simulink model "TrajectoryGenerator2DOF_freq"  (R2023b)
settings: Solver=FixedStepDiscrete  StartTime=0.0  StopTime=1.2*1.4  FixedStep=0.002  RelTol=1e-3
undefined symbols (not defined in the file or in its folder): M_z, Smoothers, Ts
(part 2 of 2)

== system TrajectoryGenerator2DOF_freq/Trajectory Generator4/M12 ==
  x : Inport
  Discrete FIR Filter1 : DiscreteFir  Coefficients=1/N/Ts*[1 zeros(1,N-1) -1]  InitialStates=Q0  SampleTime=Ts
  Discrete Filter : DiscreteFilter  Numerator=[0 Ts]  Denominator=[1 -1]  InitialStates=Q0  SampleTime=Ts
  y : Outport
  dy : Outport  Port=2
  wires:
  Discrete FIR Filter1/1 -> Discrete Filter/1, dy/1
  x/1 -> Discrete FIR Filter1/1
  Discrete Filter/1 -> y/1

== system TrajectoryGenerator2DOF_freq/Trajectory Generator4/M13 ==
  x : Inport
  Discrete FIR Filter1 : DiscreteFir  Coefficients=1/N/Ts*[1 zeros(1,N-1) -1]  InitialStates=Q0  SampleTime=Ts
  Discrete Filter : DiscreteFilter  Numerator=[0 Ts]  Denominator=[1 -1]  InitialStates=Q0  SampleTime=Ts
  y : Outport
  dy : Outport  Port=2
  wires:
  Discrete FIR Filter1/1 -> Discrete Filter/1, dy/1
  x/1 -> Discrete FIR Filter1/1
  Discrete Filter/1 -> y/1

== system TrajectoryGenerator2DOF_freq/Trajectory Generator4/M14 ==
  x : Inport
  Discrete FIR Filter1 : DiscreteFir  Coefficients=1/N/Ts*[1 zeros(1,N-1) -1]  InitialStates=Q0  SampleTime=Ts
  Discrete Filter : DiscreteFilter  Numerator=[0 Ts]  Denominator=[1 -1]  InitialStates=Q0  SampleTime=Ts
  y : Outport
  dy : Outport  Port=2
  wires:
  Discrete FIR Filter1/1 -> Discrete Filter/1, dy/1
  x/1 -> Discrete FIR Filter1/1
  Discrete Filter/1 -> y/1

== system TrajectoryGenerator2DOF_freq/Trajectory Generator4/M22 ==
  x : Inport
  Discrete FIR Filter1 : DiscreteFir  Coefficients=1/N/Ts*[1 zeros(1,N-1) -1]  InitialStates=Q0  SampleTime=Ts
  Discrete Filter : DiscreteFilter  Numerator=[0 Ts]  Denominator=[1 -1]  InitialStates=Q0  SampleTime=Ts
  y : Outport
  dy : Outport  Port=2
  wires:
  Discrete FIR Filter1/1 -> Discrete Filter/1, dy/1
  x/1 -> Discrete FIR Filter1/1
  Discrete Filter/1 -> y/1

== system TrajectoryGenerator2DOF_freq/Trajectory Generator4/M23 ==
  x : Inport
  Discrete FIR Filter1 : DiscreteFir  Coefficients=1/N/Ts*[1 zeros(1,N-1) -1]  InitialStates=Q0  SampleTime=Ts
  Discrete Filter : DiscreteFilter  Numerator=[0 Ts]  Denominator=[1 -1]  InitialStates=Q0  SampleTime=Ts
  y : Outport
  dy : Outport  Port=2
  wires:
  Discrete FIR Filter1/1 -> Discrete Filter/1, dy/1
  x/1 -> Discrete FIR Filter1/1
  Discrete Filter/1 -> y/1

== system TrajectoryGenerator2DOF_freq/Trajectory Generator4/M24 ==
  x : Inport
  Discrete FIR Filter1 : DiscreteFir  Coefficients=1/N/Ts*[1 zeros(1,N-1) -1]  InitialStates=Q0  SampleTime=Ts
  Discrete Filter : DiscreteFilter  Numerator=[0 Ts]  Denominator=[1 -1]  InitialStates=Q0  SampleTime=Ts
  y : Outport
  dy : Outport  Port=2
  wires:
  Discrete FIR Filter1/1 -> Discrete Filter/1, dy/1
  x/1 -> Discrete FIR Filter1/1
  Discrete Filter/1 -> y/1

== system TrajectoryGenerator2DOF_freq/Trajectory Generator4/M33 ==
  x : Inport
  Discrete FIR Filter1 : DiscreteFir  Coefficients=1/N/Ts*[1 zeros(1,N-1) -1]  InitialStates=Q0  SampleTime=Ts
  Discrete Filter : DiscreteFilter  Numerator=[0 Ts]  Denominator=[1 -1]  InitialStates=Q0  SampleTime=Ts
  y : Outport
  dy : Outport  Port=2
  wires:
  Discrete FIR Filter1/1 -> Discrete Filter/1, dy/1
  x/1 -> Discrete FIR Filter1/1
  Discrete Filter/1 -> y/1

== system TrajectoryGenerator2DOF_freq/Trajectory Generator4/M34 ==
  x : Inport
  Discrete FIR Filter1 : DiscreteFir  Coefficients=1/N/Ts*[1 zeros(1,N-1) -1]  InitialStates=Q0  SampleTime=Ts
  Discrete Filter : DiscreteFilter  Numerator=[0 Ts]  Denominator=[1 -1]  InitialStates=Q0  SampleTime=Ts
  y : Outport
  dy : Outport  Port=2
  wires:
  Discrete FIR Filter1/1 -> Discrete Filter/1, dy/1
  x/1 -> Discrete FIR Filter1/1
  Discrete Filter/1 -> y/1

== system TrajectoryGenerator2DOF_freq/Trajectory Generator4/M44 ==
  x : Inport
  Discrete FIR Filter1 : DiscreteFir  Coefficients=1/N/Ts*[1 zeros(1,N-1) -1]  InitialStates=Q0  SampleTime=Ts
  Discrete Filter : DiscreteFilter  Numerator=[0 Ts]  Denominator=[1 -1]  InitialStates=Q0  SampleTime=Ts
  y : Outport
  dy : Outport  Port=2
  wires:
  Discrete FIR Filter1/1 -> Discrete Filter/1, dy/1
  x/1 -> Discrete FIR Filter1/1
  Discrete Filter/1 -> y/1

== system TrajectoryGenerator2DOF_freq/Trajectory Generator5/M11 ==
  x : Inport
  Discrete FIR Filter1 : DiscreteFir  Coefficients=1/N/Ts*[1 zeros(1,N-1) -1]  InitialStates=Q0  SampleTime=Ts
  Discrete Filter : DiscreteFilter  Numerator=[0 Ts]  Denominator=[1 -1]  InitialStates=Q0  SampleTime=Ts
  y : Outport
  dy : Outport  Port=2
  wires:
  Discrete FIR Filter1/1 -> Discrete Filter/1, dy/1
  x/1 -> Discrete FIR Filter1/1
  Discrete Filter/1 -> y/1

== system TrajectoryGenerator2DOF_freq/Trajectory Generator5/M12 ==
  x : Inport
  Discrete FIR Filter1 : DiscreteFir  Coefficients=1/N/Ts*[1 zeros(1,N-1) -1]  InitialStates=Q0  SampleTime=Ts
  Discrete Filter : DiscreteFilter  Numerator=[0 Ts]  Denominator=[1 -1]  InitialStates=Q0  SampleTime=Ts
  y : Outport
  dy : Outport  Port=2
  wires:
  Discrete FIR Filter1/1 -> Discrete Filter/1, dy/1
  x/1 -> Discrete FIR Filter1/1
  Discrete Filter/1 -> y/1

== system TrajectoryGenerator2DOF_freq/Trajectory Generator5/M13 ==
  x : Inport
  Discrete FIR Filter1 : DiscreteFir  Coefficients=1/N/Ts*[1 zeros(1,N-1) -1]  InitialStates=Q0  SampleTime=Ts
  Discrete Filter : DiscreteFilter  Numerator=[0 Ts]  Denominator=[1 -1]  InitialStates=Q0  SampleTime=Ts
  y : Outport
  dy : Outport  Port=2
  wires:
  Discrete FIR Filter1/1 -> Discrete Filter/1, dy/1
  x/1 -> Discrete FIR Filter1/1
  Discrete Filter/1 -> y/1

== system TrajectoryGenerator2DOF_freq/Trajectory Generator5/M14 ==
  x : Inport
  Discrete FIR Filter1 : DiscreteFir  Coefficients=1/N/Ts*[1 zeros(1,N-1) -1]  InitialStates=Q0  SampleTime=Ts
  Discrete Filter : DiscreteFilter  Numerator=[0 Ts]  Denominator=[1 -1]  InitialStates=Q0  SampleTime=Ts
  y : Outport
  dy : Outport  Port=2
  wires:
  Discrete FIR Filter1/1 -> Discrete Filter/1, dy/1
  x/1 -> Discrete FIR Filter1/1
  Discrete Filter/1 -> y/1

== system TrajectoryGenerator2DOF_freq/Trajectory Generator5/M22 ==
  x : Inport
  Discrete FIR Filter1 : DiscreteFir  Coefficients=1/N/Ts*[1 zeros(1,N-1) -1]  InitialStates=Q0  SampleTime=Ts
  Discrete Filter : DiscreteFilter  Numerator=[0 Ts]  Denominator=[1 -1]  InitialStates=Q0  SampleTime=Ts
  y : Outport
  dy : Outport  Port=2
  wires:
  Discrete FIR Filter1/1 -> Discrete Filter/1, dy/1
  x/1 -> Discrete FIR Filter1/1
  Discrete Filter/1 -> y/1

== system TrajectoryGenerator2DOF_freq/Trajectory Generator5/M23 ==
  x : Inport
  Discrete FIR Filter1 : DiscreteFir  Coefficients=1/N/Ts*[1 zeros(1,N-1) -1]  InitialStates=Q0  SampleTime=Ts
  Discrete Filter : DiscreteFilter  Numerator=[0 Ts]  Denominator=[1 -1]  InitialStates=Q0  SampleTime=Ts
  y : Outport
  dy : Outport  Port=2
  wires:
  Discrete FIR Filter1/1 -> Discrete Filter/1, dy/1
  x/1 -> Discrete FIR Filter1/1
  Discrete Filter/1 -> y/1

== system TrajectoryGenerator2DOF_freq/Trajectory Generator5/M24 ==
  x : Inport
  Discrete FIR Filter1 : DiscreteFir  Coefficients=1/N/Ts*[1 zeros(1,N-1) -1]  InitialStates=Q0  SampleTime=Ts
  Discrete Filter : DiscreteFilter  Numerator=[0 Ts]  Denominator=[1 -1]  InitialStates=Q0  SampleTime=Ts
  y : Outport
  dy : Outport  Port=2
  wires:
  Discrete FIR Filter1/1 -> Discrete Filter/1, dy/1
  x/1 -> Discrete FIR Filter1/1
  Discrete Filter/1 -> y/1

== system TrajectoryGenerator2DOF_freq/Trajectory Generator5/M33 ==
  x : Inport
  Discrete FIR Filter1 : DiscreteFir  Coefficients=1/N/Ts*[1 zeros(1,N-1) -1]  InitialStates=Q0  SampleTime=Ts
  Discrete Filter : DiscreteFilter  Numerator=[0 Ts]  Denominator=[1 -1]  InitialStates=Q0  SampleTime=Ts
  y : Outport
  dy : Outport  Port=2
  wires:
  Discrete FIR Filter1/1 -> Discrete Filter/1, dy/1
  x/1 -> Discrete FIR Filter1/1
  Discrete Filter/1 -> y/1

== system TrajectoryGenerator2DOF_freq/Trajectory Generator5/M34 ==
  x : Inport
  Discrete FIR Filter1 : DiscreteFir  Coefficients=1/N/Ts*[1 zeros(1,N-1) -1]  InitialStates=Q0  SampleTime=Ts
  Discrete Filter : DiscreteFilter  Numerator=[0 Ts]  Denominator=[1 -1]  InitialStates=Q0  SampleTime=Ts
  y : Outport
  dy : Outport  Port=2
  wires:
  Discrete FIR Filter1/1 -> Discrete Filter/1, dy/1
  x/1 -> Discrete FIR Filter1/1
  Discrete Filter/1 -> y/1

== system TrajectoryGenerator2DOF_freq/Trajectory Generator5/M44 ==
  x : Inport
  Discrete FIR Filter1 : DiscreteFir  Coefficients=1/N/Ts*[1 zeros(1,N-1) -1]  InitialStates=Q0  SampleTime=Ts
  Discrete Filter : DiscreteFilter  Numerator=[0 Ts]  Denominator=[1 -1]  InitialStates=Q0  SampleTime=Ts
  y : Outport
  dy : Outport  Port=2
  wires:
  Discrete FIR Filter1/1 -> Discrete Filter/1, dy/1
  x/1 -> Discrete FIR Filter1/1
  Discrete Filter/1 -> y/1

== system TrajectoryGenerator2DOF_freq/Trajectory Generator6/M11 ==
  x : Inport
  Discrete FIR Filter1 : DiscreteFir  Coefficients=1/N/Ts*[1 zeros(1,N-1) -1]  InitialStates=Q0  SampleTime=Ts
  Discrete Filter : DiscreteFilter  Numerator=[0 Ts]  Denominator=[1 -1]  InitialStates=Q0  SampleTime=Ts
  y : Outport
  dy : Outport  Port=2
  wires:
  Discrete FIR Filter1/1 -> Discrete Filter/1, dy/1
  x/1 -> Discrete FIR Filter1/1
  Discrete Filter/1 -> y/1

== system TrajectoryGenerator2DOF_freq/Trajectory Generator6/M12 ==
  x : Inport
  Discrete FIR Filter1 : DiscreteFir  Coefficients=1/N/Ts*[1 zeros(1,N-1) -1]  InitialStates=Q0  SampleTime=Ts
  Discrete Filter : DiscreteFilter  Numerator=[0 Ts]  Denominator=[1 -1]  InitialStates=Q0  SampleTime=Ts
  y : Outport
  dy : Outport  Port=2
  wires:
  Discrete FIR Filter1/1 -> Discrete Filter/1, dy/1
  x/1 -> Discrete FIR Filter1/1
  Discrete Filter/1 -> y/1

== system TrajectoryGenerator2DOF_freq/Trajectory Generator6/M13 ==
  x : Inport
  Discrete FIR Filter1 : DiscreteFir  Coefficients=1/N/Ts*[1 zeros(1,N-1) -1]  InitialStates=Q0  SampleTime=Ts
  Discrete Filter : DiscreteFilter  Numerator=[0 Ts]  Denominator=[1 -1]  InitialStates=Q0  SampleTime=Ts
  y : Outport
  dy : Outport  Port=2
  wires:
  Discrete FIR Filter1/1 -> Discrete Filter/1, dy/1
  x/1 -> Discrete FIR Filter1/1
  Discrete Filter/1 -> y/1

== system TrajectoryGenerator2DOF_freq/Trajectory Generator6/M14 ==
  x : Inport
  Discrete FIR Filter1 : DiscreteFir  Coefficients=1/N/Ts*[1 zeros(1,N-1) -1]  InitialStates=Q0  SampleTime=Ts
  Discrete Filter : DiscreteFilter  Numerator=[0 Ts]  Denominator=[1 -1]  InitialStates=Q0  SampleTime=Ts
  y : Outport
  dy : Outport  Port=2
  wires:
  Discrete FIR Filter1/1 -> Discrete Filter/1, dy/1
  x/1 -> Discrete FIR Filter1/1
  Discrete Filter/1 -> y/1

== system TrajectoryGenerator2DOF_freq/Trajectory Generator6/M22 ==
  x : Inport
  Discrete FIR Filter1 : DiscreteFir  Coefficients=1/N/Ts*[1 zeros(1,N-1) -1]  InitialStates=Q0  SampleTime=Ts
  Discrete Filter : DiscreteFilter  Numerator=[0 Ts]  Denominator=[1 -1]  InitialStates=Q0  SampleTime=Ts
  y : Outport
  dy : Outport  Port=2
  wires:
  Discrete FIR Filter1/1 -> Discrete Filter/1, dy/1
  x/1 -> Discrete FIR Filter1/1
  Discrete Filter/1 -> y/1

== system TrajectoryGenerator2DOF_freq/Trajectory Generator6/M23 ==
  x : Inport
  Discrete FIR Filter1 : DiscreteFir  Coefficients=1/N/Ts*[1 zeros(1,N-1) -1]  InitialStates=Q0  SampleTime=Ts
  Discrete Filter : DiscreteFilter  Numerator=[0 Ts]  Denominator=[1 -1]  InitialStates=Q0  SampleTime=Ts
  y : Outport
  dy : Outport  Port=2
  wires:
  Discrete FIR Filter1/1 -> Discrete Filter/1, dy/1
  x/1 -> Discrete FIR Filter1/1
  Discrete Filter/1 -> y/1

== system TrajectoryGenerator2DOF_freq/Trajectory Generator6/M24 ==
  x : Inport
  Discrete FIR Filter1 : DiscreteFir  Coefficients=1/N/Ts*[1 zeros(1,N-1) -1]  InitialStates=Q0  SampleTime=Ts
  Discrete Filter : DiscreteFilter  Numerator=[0 Ts]  Denominator=[1 -1]  InitialStates=Q0  SampleTime=Ts
  y : Outport
  dy : Outport  Port=2
  wires:
  Discrete FIR Filter1/1 -> Discrete Filter/1, dy/1
  x/1 -> Discrete FIR Filter1/1
  Discrete Filter/1 -> y/1

== system TrajectoryGenerator2DOF_freq/Trajectory Generator6/M33 ==
  x : Inport
  Discrete FIR Filter1 : DiscreteFir  Coefficients=1/N/Ts*[1 zeros(1,N-1) -1]  InitialStates=Q0  SampleTime=Ts
  Discrete Filter : DiscreteFilter  Numerator=[0 Ts]  Denominator=[1 -1]  InitialStates=Q0  SampleTime=Ts
  y : Outport
  dy : Outport  Port=2
  wires:
  Discrete FIR Filter1/1 -> Discrete Filter/1, dy/1
  x/1 -> Discrete FIR Filter1/1
  Discrete Filter/1 -> y/1

== system TrajectoryGenerator2DOF_freq/Trajectory Generator6/M34 ==
  x : Inport
  Discrete FIR Filter1 : DiscreteFir  Coefficients=1/N/Ts*[1 zeros(1,N-1) -1]  InitialStates=Q0  SampleTime=Ts
  Discrete Filter : DiscreteFilter  Numerator=[0 Ts]  Denominator=[1 -1]  InitialStates=Q0  SampleTime=Ts
  y : Outport
  dy : Outport  Port=2
  wires:
  Discrete FIR Filter1/1 -> Discrete Filter/1, dy/1
  x/1 -> Discrete FIR Filter1/1
  Discrete Filter/1 -> y/1

== system TrajectoryGenerator2DOF_freq/Trajectory Generator6/M44 ==
  x : Inport
  Discrete FIR Filter1 : DiscreteFir  Coefficients=1/N/Ts*[1 zeros(1,N-1) -1]  InitialStates=Q0  SampleTime=Ts
  Discrete Filter : DiscreteFilter  Numerator=[0 Ts]  Denominator=[1 -1]  InitialStates=Q0  SampleTime=Ts
  y : Outport
  dy : Outport  Port=2
  wires:
  Discrete FIR Filter1/1 -> Discrete Filter/1, dy/1
  x/1 -> Discrete FIR Filter1/1
  Discrete Filter/1 -> y/1

== system TrajectoryGenerator2DOF_freq/Trajectory Generator7/M11 ==
  x : Inport
  Discrete FIR Filter1 : DiscreteFir  Coefficients=1/N/Ts*[1 zeros(1,N-1) -1]  InitialStates=Q0  SampleTime=Ts
  Discrete Filter : DiscreteFilter  Numerator=[0 Ts]  Denominator=[1 -1]  InitialStates=Q0  SampleTime=Ts
  y : Outport
  dy : Outport  Port=2
  wires:
  Discrete FIR Filter1/1 -> Discrete Filter/1, dy/1
  x/1 -> Discrete FIR Filter1/1
  Discrete Filter/1 -> y/1

== system TrajectoryGenerator2DOF_freq/Trajectory Generator7/M12 ==
  x : Inport
  Discrete FIR Filter1 : DiscreteFir  Coefficients=1/N/Ts*[1 zeros(1,N-1) -1]  InitialStates=Q0  SampleTime=Ts
  Discrete Filter : DiscreteFilter  Numerator=[0 Ts]  Denominator=[1 -1]  InitialStates=Q0  SampleTime=Ts
  y : Outport
  dy : Outport  Port=2
  wires:
  Discrete FIR Filter1/1 -> Discrete Filter/1, dy/1
  x/1 -> Discrete FIR Filter1/1
  Discrete Filter/1 -> y/1

== system TrajectoryGenerator2DOF_freq/Trajectory Generator7/M13 ==
  x : Inport
  Discrete FIR Filter1 : DiscreteFir  Coefficients=1/N/Ts*[1 zeros(1,N-1) -1]  InitialStates=Q0  SampleTime=Ts
  Discrete Filter : DiscreteFilter  Numerator=[0 Ts]  Denominator=[1 -1]  InitialStates=Q0  SampleTime=Ts
  y : Outport
  dy : Outport  Port=2
  wires:
  Discrete FIR Filter1/1 -> Discrete Filter/1, dy/1
  x/1 -> Discrete FIR Filter1/1
  Discrete Filter/1 -> y/1

== system TrajectoryGenerator2DOF_freq/Trajectory Generator7/M14 ==
  x : Inport
  Discrete FIR Filter1 : DiscreteFir  Coefficients=1/N/Ts*[1 zeros(1,N-1) -1]  InitialStates=Q0  SampleTime=Ts
  Discrete Filter : DiscreteFilter  Numerator=[0 Ts]  Denominator=[1 -1]  InitialStates=Q0  SampleTime=Ts
  y : Outport
  dy : Outport  Port=2
  wires:
  Discrete FIR Filter1/1 -> Discrete Filter/1, dy/1
  x/1 -> Discrete FIR Filter1/1
  Discrete Filter/1 -> y/1

== system TrajectoryGenerator2DOF_freq/Trajectory Generator7/M22 ==
  x : Inport
  Discrete FIR Filter1 : DiscreteFir  Coefficients=1/N/Ts*[1 zeros(1,N-1) -1]  InitialStates=Q0  SampleTime=Ts
  Discrete Filter : DiscreteFilter  Numerator=[0 Ts]  Denominator=[1 -1]  InitialStates=Q0  SampleTime=Ts
  y : Outport
  dy : Outport  Port=2
  wires:
  Discrete FIR Filter1/1 -> Discrete Filter/1, dy/1
  x/1 -> Discrete FIR Filter1/1
  Discrete Filter/1 -> y/1

== system TrajectoryGenerator2DOF_freq/Trajectory Generator7/M23 ==
  x : Inport
  Discrete FIR Filter1 : DiscreteFir  Coefficients=1/N/Ts*[1 zeros(1,N-1) -1]  InitialStates=Q0  SampleTime=Ts
  Discrete Filter : DiscreteFilter  Numerator=[0 Ts]  Denominator=[1 -1]  InitialStates=Q0  SampleTime=Ts
  y : Outport
  dy : Outport  Port=2
  wires:
  Discrete FIR Filter1/1 -> Discrete Filter/1, dy/1
  x/1 -> Discrete FIR Filter1/1
  Discrete Filter/1 -> y/1

== system TrajectoryGenerator2DOF_freq/Trajectory Generator7/M24 ==
  x : Inport
  Discrete FIR Filter1 : DiscreteFir  Coefficients=1/N/Ts*[1 zeros(1,N-1) -1]  InitialStates=Q0  SampleTime=Ts
  Discrete Filter : DiscreteFilter  Numerator=[0 Ts]  Denominator=[1 -1]  InitialStates=Q0  SampleTime=Ts
  y : Outport
  dy : Outport  Port=2
  wires:
  Discrete FIR Filter1/1 -> Discrete Filter/1, dy/1
  x/1 -> Discrete FIR Filter1/1
  Discrete Filter/1 -> y/1

== system TrajectoryGenerator2DOF_freq/Trajectory Generator7/M33 ==
  x : Inport
  Discrete FIR Filter1 : DiscreteFir  Coefficients=1/N/Ts*[1 zeros(1,N-1) -1]  InitialStates=Q0  SampleTime=Ts
  Discrete Filter : DiscreteFilter  Numerator=[0 Ts]  Denominator=[1 -1]  InitialStates=Q0  SampleTime=Ts
  y : Outport
  dy : Outport  Port=2
  wires:
  Discrete FIR Filter1/1 -> Discrete Filter/1, dy/1
  x/1 -> Discrete FIR Filter1/1
  Discrete Filter/1 -> y/1

== system TrajectoryGenerator2DOF_freq/Trajectory Generator7/M34 ==
  x : Inport
  Discrete FIR Filter1 : DiscreteFir  Coefficients=1/N/Ts*[1 zeros(1,N-1) -1]  InitialStates=Q0  SampleTime=Ts
  Discrete Filter : DiscreteFilter  Numerator=[0 Ts]  Denominator=[1 -1]  InitialStates=Q0  SampleTime=Ts
  y : Outport
  dy : Outport  Port=2
  wires:
  Discrete FIR Filter1/1 -> Discrete Filter/1, dy/1
  x/1 -> Discrete FIR Filter1/1
  Discrete Filter/1 -> y/1

== system TrajectoryGenerator2DOF_freq/Trajectory Generator7/M44 ==
  x : Inport
  Discrete FIR Filter1 : DiscreteFir  Coefficients=1/N/Ts*[1 zeros(1,N-1) -1]  InitialStates=Q0  SampleTime=Ts
  Discrete Filter : DiscreteFilter  Numerator=[0 Ts]  Denominator=[1 -1]  InitialStates=Q0  SampleTime=Ts
  y : Outport
  dy : Outport  Port=2
  wires:
  Discrete FIR Filter1/1 -> Discrete Filter/1, dy/1
  x/1 -> Discrete FIR Filter1/1
  Discrete Filter/1 -> y/1

== system TrajectoryGenerator2DOF_freq/Trajectory Generator8/M11 ==
  x : Inport
  Discrete FIR Filter1 : DiscreteFir  Coefficients=1/N/Ts*[1 zeros(1,N-1) -1]  InitialStates=Q0  SampleTime=Ts
  Discrete Filter : DiscreteFilter  Numerator=[0 Ts]  Denominator=[1 -1]  InitialStates=Q0  SampleTime=Ts
  y : Outport
  dy : Outport  Port=2
  wires:
  Discrete FIR Filter1/1 -> Discrete Filter/1, dy/1
  x/1 -> Discrete FIR Filter1/1
  Discrete Filter/1 -> y/1

== system TrajectoryGenerator2DOF_freq/Trajectory Generator8/M12 ==
  x : Inport
  Discrete FIR Filter1 : DiscreteFir  Coefficients=1/N/Ts*[1 zeros(1,N-1) -1]  InitialStates=Q0  SampleTime=Ts
  Discrete Filter : DiscreteFilter  Numerator=[0 Ts]  Denominator=[1 -1]  InitialStates=Q0  SampleTime=Ts
  y : Outport
  dy : Outport  Port=2
  wires:
  Discrete FIR Filter1/1 -> Discrete Filter/1, dy/1
  x/1 -> Discrete FIR Filter1/1
  Discrete Filter/1 -> y/1

== system TrajectoryGenerator2DOF_freq/Trajectory Generator8/M13 ==
  x : Inport
  Discrete FIR Filter1 : DiscreteFir  Coefficients=1/N/Ts*[1 zeros(1,N-1) -1]  InitialStates=Q0  SampleTime=Ts
  Discrete Filter : DiscreteFilter  Numerator=[0 Ts]  Denominator=[1 -1]  InitialStates=Q0  SampleTime=Ts
  y : Outport
  dy : Outport  Port=2
  wires:
  Discrete FIR Filter1/1 -> Discrete Filter/1, dy/1
  x/1 -> Discrete FIR Filter1/1
  Discrete Filter/1 -> y/1

== system TrajectoryGenerator2DOF_freq/Trajectory Generator8/M14 ==
  x : Inport
  Discrete FIR Filter1 : DiscreteFir  Coefficients=1/N/Ts*[1 zeros(1,N-1) -1]  InitialStates=Q0  SampleTime=Ts
  Discrete Filter : DiscreteFilter  Numerator=[0 Ts]  Denominator=[1 -1]  InitialStates=Q0  SampleTime=Ts
  y : Outport
  dy : Outport  Port=2
  wires:
  Discrete FIR Filter1/1 -> Discrete Filter/1, dy/1
  x/1 -> Discrete FIR Filter1/1
  Discrete Filter/1 -> y/1

== system TrajectoryGenerator2DOF_freq/Trajectory Generator8/M15 ==
  x : Inport
  Discrete FIR Filter1 : DiscreteFir  Coefficients=1/N/Ts*[1 zeros(1,N-1) -1]  InitialStates=Q0  SampleTime=Ts
  Discrete Filter : DiscreteFilter  Numerator=[0 Ts]  Denominator=[1 -1]  InitialStates=Q0  SampleTime=Ts
  y : Outport
  dy : Outport  Port=2
  wires:
  Discrete FIR Filter1/1 -> Discrete Filter/1, dy/1
  x/1 -> Discrete FIR Filter1/1
  Discrete Filter/1 -> y/1

== system TrajectoryGenerator2DOF_freq/Trajectory Generator8/M16 ==
  x : Inport
  Discrete FIR Filter1 : DiscreteFir  Coefficients=1/N/Ts*[1 zeros(1,N-1) -1]  InitialStates=Q0  SampleTime=Ts
  Discrete Filter : DiscreteFilter  Numerator=[0 Ts]  Denominator=[1 -1]  InitialStates=Q0  SampleTime=Ts
  y : Outport
  dy : Outport  Port=2
  wires:
  Discrete FIR Filter1/1 -> Discrete Filter/1, dy/1
  x/1 -> Discrete FIR Filter1/1
  Discrete Filter/1 -> y/1

== system TrajectoryGenerator2DOF_freq/Trajectory Generator8/M22 ==
  x : Inport
  Discrete FIR Filter1 : DiscreteFir  Coefficients=1/N/Ts*[1 zeros(1,N-1) -1]  InitialStates=Q0  SampleTime=Ts
  Discrete Filter : DiscreteFilter  Numerator=[0 Ts]  Denominator=[1 -1]  InitialStates=Q0  SampleTime=Ts
  y : Outport
  dy : Outport  Port=2
  wires:
  Discrete FIR Filter1/1 -> Discrete Filter/1, dy/1
  x/1 -> Discrete FIR Filter1/1
  Discrete Filter/1 -> y/1

== system TrajectoryGenerator2DOF_freq/Trajectory Generator8/M23 ==
  x : Inport
  Discrete FIR Filter1 : DiscreteFir  Coefficients=1/N/Ts*[1 zeros(1,N-1) -1]  InitialStates=Q0  SampleTime=Ts
  Discrete Filter : DiscreteFilter  Numerator=[0 Ts]  Denominator=[1 -1]  InitialStates=Q0  SampleTime=Ts
  y : Outport
  dy : Outport  Port=2
  wires:
  Discrete FIR Filter1/1 -> Discrete Filter/1, dy/1
  x/1 -> Discrete FIR Filter1/1
  Discrete Filter/1 -> y/1

== system TrajectoryGenerator2DOF_freq/Trajectory Generator8/M24 ==
  x : Inport
  Discrete FIR Filter1 : DiscreteFir  Coefficients=1/N/Ts*[1 zeros(1,N-1) -1]  InitialStates=Q0  SampleTime=Ts
  Discrete Filter : DiscreteFilter  Numerator=[0 Ts]  Denominator=[1 -1]  InitialStates=Q0  SampleTime=Ts
  y : Outport
  dy : Outport  Port=2
  wires:
  Discrete FIR Filter1/1 -> Discrete Filter/1, dy/1
  x/1 -> Discrete FIR Filter1/1
  Discrete Filter/1 -> y/1

== system TrajectoryGenerator2DOF_freq/Trajectory Generator8/M25 ==
  x : Inport
  Discrete FIR Filter1 : DiscreteFir  Coefficients=1/N/Ts*[1 zeros(1,N-1) -1]  InitialStates=Q0  SampleTime=Ts
  Discrete Filter : DiscreteFilter  Numerator=[0 Ts]  Denominator=[1 -1]  InitialStates=Q0  SampleTime=Ts
  y : Outport
  dy : Outport  Port=2
  wires:
  Discrete FIR Filter1/1 -> Discrete Filter/1, dy/1
  x/1 -> Discrete FIR Filter1/1
  Discrete Filter/1 -> y/1

== system TrajectoryGenerator2DOF_freq/Trajectory Generator8/M26 ==
  x : Inport
  Discrete FIR Filter1 : DiscreteFir  Coefficients=1/N/Ts*[1 zeros(1,N-1) -1]  InitialStates=Q0  SampleTime=Ts
  Discrete Filter : DiscreteFilter  Numerator=[0 Ts]  Denominator=[1 -1]  InitialStates=Q0  SampleTime=Ts
  y : Outport
  dy : Outport  Port=2
  wires:
  Discrete FIR Filter1/1 -> Discrete Filter/1, dy/1
  x/1 -> Discrete FIR Filter1/1
  Discrete Filter/1 -> y/1

== system TrajectoryGenerator2DOF_freq/Trajectory Generator8/M33 ==
  x : Inport
  Discrete FIR Filter1 : DiscreteFir  Coefficients=1/N/Ts*[1 zeros(1,N-1) -1]  InitialStates=Q0  SampleTime=Ts
  Discrete Filter : DiscreteFilter  Numerator=[0 Ts]  Denominator=[1 -1]  InitialStates=Q0  SampleTime=Ts
  y : Outport
  dy : Outport  Port=2
  wires:
  Discrete FIR Filter1/1 -> Discrete Filter/1, dy/1
  x/1 -> Discrete FIR Filter1/1
  Discrete Filter/1 -> y/1

== system TrajectoryGenerator2DOF_freq/Trajectory Generator8/M34 ==
  x : Inport
  Discrete FIR Filter1 : DiscreteFir  Coefficients=1/N/Ts*[1 zeros(1,N-1) -1]  InitialStates=Q0  SampleTime=Ts
  Discrete Filter : DiscreteFilter  Numerator=[0 Ts]  Denominator=[1 -1]  InitialStates=Q0  SampleTime=Ts
  y : Outport
  dy : Outport  Port=2
  wires:
  Discrete FIR Filter1/1 -> Discrete Filter/1, dy/1
  x/1 -> Discrete FIR Filter1/1
  Discrete Filter/1 -> y/1

== system TrajectoryGenerator2DOF_freq/Trajectory Generator8/M35 ==
  x : Inport
  Discrete FIR Filter1 : DiscreteFir  Coefficients=1/N/Ts*[1 zeros(1,N-1) -1]  InitialStates=Q0  SampleTime=Ts
  Discrete Filter : DiscreteFilter  Numerator=[0 Ts]  Denominator=[1 -1]  InitialStates=Q0  SampleTime=Ts
  y : Outport
  dy : Outport  Port=2
  wires:
  Discrete FIR Filter1/1 -> Discrete Filter/1, dy/1
  x/1 -> Discrete FIR Filter1/1
  Discrete Filter/1 -> y/1

== system TrajectoryGenerator2DOF_freq/Trajectory Generator8/M36 ==
  x : Inport
  Discrete FIR Filter1 : DiscreteFir  Coefficients=1/N/Ts*[1 zeros(1,N-1) -1]  InitialStates=Q0  SampleTime=Ts
  Discrete Filter : DiscreteFilter  Numerator=[0 Ts]  Denominator=[1 -1]  InitialStates=Q0  SampleTime=Ts
  y : Outport
  dy : Outport  Port=2
  wires:
  Discrete FIR Filter1/1 -> Discrete Filter/1, dy/1
  x/1 -> Discrete FIR Filter1/1
  Discrete Filter/1 -> y/1

== system TrajectoryGenerator2DOF_freq/Trajectory Generator8/M44 ==
  x : Inport
  Discrete FIR Filter1 : DiscreteFir  Coefficients=1/N/Ts*[1 zeros(1,N-1) -1]  InitialStates=Q0  SampleTime=Ts
  Discrete Filter : DiscreteFilter  Numerator=[0 Ts]  Denominator=[1 -1]  InitialStates=Q0  SampleTime=Ts
  y : Outport
  dy : Outport  Port=2
  wires:
  Discrete FIR Filter1/1 -> Discrete Filter/1, dy/1
  x/1 -> Discrete FIR Filter1/1
  Discrete Filter/1 -> y/1

== system TrajectoryGenerator2DOF_freq/Trajectory Generator8/M45 ==
  x : Inport
  Discrete FIR Filter1 : DiscreteFir  Coefficients=1/N/Ts*[1 zeros(1,N-1) -1]  InitialStates=Q0  SampleTime=Ts
  Discrete Filter : DiscreteFilter  Numerator=[0 Ts]  Denominator=[1 -1]  InitialStates=Q0  SampleTime=Ts
  y : Outport
  dy : Outport  Port=2
  wires:
  Discrete FIR Filter1/1 -> Discrete Filter/1, dy/1
  x/1 -> Discrete FIR Filter1/1
  Discrete Filter/1 -> y/1

== system TrajectoryGenerator2DOF_freq/Trajectory Generator8/M46 ==
  x : Inport
  Discrete FIR Filter1 : DiscreteFir  Coefficients=1/N/Ts*[1 zeros(1,N-1) -1]  InitialStates=Q0  SampleTime=Ts
  Discrete Filter : DiscreteFilter  Numerator=[0 Ts]  Denominator=[1 -1]  InitialStates=Q0  SampleTime=Ts
  y : Outport
  dy : Outport  Port=2
  wires:
  Discrete FIR Filter1/1 -> Discrete Filter/1, dy/1
  x/1 -> Discrete FIR Filter1/1
  Discrete Filter/1 -> y/1

== system TrajectoryGenerator2DOF_freq/Trajectory Generator8/M55 ==
  x : Inport
  Discrete FIR Filter1 : DiscreteFir  Coefficients=1/N/Ts*[1 zeros(1,N-1) -1]  InitialStates=Q0  SampleTime=Ts
  Discrete Filter : DiscreteFilter  Numerator=[0 Ts]  Denominator=[1 -1]  InitialStates=Q0  SampleTime=Ts
  y : Outport
  dy : Outport  Port=2
  wires:
  Discrete FIR Filter1/1 -> Discrete Filter/1, dy/1
  x/1 -> Discrete FIR Filter1/1
  Discrete Filter/1 -> y/1

== system TrajectoryGenerator2DOF_freq/Trajectory Generator8/M56 ==
  x : Inport
  Discrete FIR Filter1 : DiscreteFir  Coefficients=1/N/Ts*[1 zeros(1,N-1) -1]  InitialStates=Q0  SampleTime=Ts
  Discrete Filter : DiscreteFilter  Numerator=[0 Ts]  Denominator=[1 -1]  InitialStates=Q0  SampleTime=Ts
  y : Outport
  dy : Outport  Port=2
  wires:
  Discrete FIR Filter1/1 -> Discrete Filter/1, dy/1
  x/1 -> Discrete FIR Filter1/1
  Discrete Filter/1 -> y/1

== system TrajectoryGenerator2DOF_freq/Trajectory Generator8/M66 ==
  x : Inport
  Discrete FIR Filter1 : DiscreteFir  Coefficients=1/N/Ts*[1 zeros(1,N-1) -1]  InitialStates=Q0  SampleTime=Ts
  Discrete Filter : DiscreteFilter  Numerator=[0 Ts]  Denominator=[1 -1]  InitialStates=Q0  SampleTime=Ts
  y : Outport
  dy : Outport  Port=2
  wires:
  Discrete FIR Filter1/1 -> Discrete Filter/1, dy/1
  x/1 -> Discrete FIR Filter1/1
  Discrete Filter/1 -> y/1

== system TrajectoryGenerator2DOF_freq/Trajectory Generator9/M11 ==
  x : Inport
  Discrete FIR Filter1 : DiscreteFir  Coefficients=1/N/Ts*[1 zeros(1,N-1) -1]  InitialStates=Q0  SampleTime=Ts
  Discrete Filter : DiscreteFilter  Numerator=[0 Ts]  Denominator=[1 -1]  InitialStates=Q0  SampleTime=Ts
  y : Outport
  dy : Outport  Port=2
  wires:
  Discrete FIR Filter1/1 -> Discrete Filter/1, dy/1
  x/1 -> Discrete FIR Filter1/1
  Discrete Filter/1 -> y/1

== system TrajectoryGenerator2DOF_freq/Trajectory Generator9/M12 ==
  x : Inport
  Discrete FIR Filter1 : DiscreteFir  Coefficients=1/N/Ts*[1 zeros(1,N-1) -1]  InitialStates=Q0  SampleTime=Ts
  Discrete Filter : DiscreteFilter  Numerator=[0 Ts]  Denominator=[1 -1]  InitialStates=Q0  SampleTime=Ts
  y : Outport
  dy : Outport  Port=2
  wires:
  Discrete FIR Filter1/1 -> Discrete Filter/1, dy/1
  x/1 -> Discrete FIR Filter1/1
  Discrete Filter/1 -> y/1

== system TrajectoryGenerator2DOF_freq/Trajectory Generator9/M13 ==
  x : Inport
  Discrete FIR Filter1 : DiscreteFir  Coefficients=1/N/Ts*[1 zeros(1,N-1) -1]  InitialStates=Q0  SampleTime=Ts
  Discrete Filter : DiscreteFilter  Numerator=[0 Ts]  Denominator=[1 -1]  InitialStates=Q0  SampleTime=Ts
  y : Outport
  dy : Outport  Port=2
  wires:
  Discrete FIR Filter1/1 -> Discrete Filter/1, dy/1
  x/1 -> Discrete FIR Filter1/1
  Discrete Filter/1 -> y/1

== system TrajectoryGenerator2DOF_freq/Trajectory Generator9/M14 ==
  x : Inport
  Discrete FIR Filter1 : DiscreteFir  Coefficients=1/N/Ts*[1 zeros(1,N-1) -1]  InitialStates=Q0  SampleTime=Ts
  Discrete Filter : DiscreteFilter  Numerator=[0 Ts]  Denominator=[1 -1]  InitialStates=Q0  SampleTime=Ts
  y : Outport
  dy : Outport  Port=2
  wires:
  Discrete FIR Filter1/1 -> Discrete Filter/1, dy/1
  x/1 -> Discrete FIR Filter1/1
  Discrete Filter/1 -> y/1

== system TrajectoryGenerator2DOF_freq/Trajectory Generator9/M15 ==
  x : Inport
  Discrete FIR Filter1 : DiscreteFir  Coefficients=1/N/Ts*[1 zeros(1,N-1) -1]  InitialStates=Q0  SampleTime=Ts
  Discrete Filter : DiscreteFilter  Numerator=[0 Ts]  Denominator=[1 -1]  InitialStates=Q0  SampleTime=Ts
  y : Outport
  dy : Outport  Port=2
  wires:
  Discrete FIR Filter1/1 -> Discrete Filter/1, dy/1
  x/1 -> Discrete FIR Filter1/1
  Discrete Filter/1 -> y/1

== system TrajectoryGenerator2DOF_freq/Trajectory Generator9/M16 ==
  x : Inport
  Discrete FIR Filter1 : DiscreteFir  Coefficients=1/N/Ts*[1 zeros(1,N-1) -1]  InitialStates=Q0  SampleTime=Ts
  Discrete Filter : DiscreteFilter  Numerator=[0 Ts]  Denominator=[1 -1]  InitialStates=Q0  SampleTime=Ts
  y : Outport
  dy : Outport  Port=2
  wires:
  Discrete FIR Filter1/1 -> Discrete Filter/1, dy/1
  x/1 -> Discrete FIR Filter1/1
  Discrete Filter/1 -> y/1

== system TrajectoryGenerator2DOF_freq/Trajectory Generator9/M22 ==
  x : Inport
  Discrete FIR Filter1 : DiscreteFir  Coefficients=1/N/Ts*[1 zeros(1,N-1) -1]  InitialStates=Q0  SampleTime=Ts
  Discrete Filter : DiscreteFilter  Numerator=[0 Ts]  Denominator=[1 -1]  InitialStates=Q0  SampleTime=Ts
  y : Outport
  dy : Outport  Port=2
  wires:
  Discrete FIR Filter1/1 -> Discrete Filter/1, dy/1
  x/1 -> Discrete FIR Filter1/1
  Discrete Filter/1 -> y/1

== system TrajectoryGenerator2DOF_freq/Trajectory Generator9/M23 ==
  x : Inport
  Discrete FIR Filter1 : DiscreteFir  Coefficients=1/N/Ts*[1 zeros(1,N-1) -1]  InitialStates=Q0  SampleTime=Ts
  Discrete Filter : DiscreteFilter  Numerator=[0 Ts]  Denominator=[1 -1]  InitialStates=Q0  SampleTime=Ts
  y : Outport
  dy : Outport  Port=2
  wires:
  Discrete FIR Filter1/1 -> Discrete Filter/1, dy/1
  x/1 -> Discrete FIR Filter1/1
  Discrete Filter/1 -> y/1

== system TrajectoryGenerator2DOF_freq/Trajectory Generator9/M24 ==
  x : Inport
  Discrete FIR Filter1 : DiscreteFir  Coefficients=1/N/Ts*[1 zeros(1,N-1) -1]  InitialStates=Q0  SampleTime=Ts
  Discrete Filter : DiscreteFilter  Numerator=[0 Ts]  Denominator=[1 -1]  InitialStates=Q0  SampleTime=Ts
  y : Outport
  dy : Outport  Port=2
  wires:
  Discrete FIR Filter1/1 -> Discrete Filter/1, dy/1
  x/1 -> Discrete FIR Filter1/1
  Discrete Filter/1 -> y/1

== system TrajectoryGenerator2DOF_freq/Trajectory Generator9/M25 ==
  x : Inport
  Discrete FIR Filter1 : DiscreteFir  Coefficients=1/N/Ts*[1 zeros(1,N-1) -1]  InitialStates=Q0  SampleTime=Ts
  Discrete Filter : DiscreteFilter  Numerator=[0 Ts]  Denominator=[1 -1]  InitialStates=Q0  SampleTime=Ts
  y : Outport
  dy : Outport  Port=2
  wires:
  Discrete FIR Filter1/1 -> Discrete Filter/1, dy/1
  x/1 -> Discrete FIR Filter1/1
  Discrete Filter/1 -> y/1

== system TrajectoryGenerator2DOF_freq/Trajectory Generator9/M26 ==
  x : Inport
  Discrete FIR Filter1 : DiscreteFir  Coefficients=1/N/Ts*[1 zeros(1,N-1) -1]  InitialStates=Q0  SampleTime=Ts
  Discrete Filter : DiscreteFilter  Numerator=[0 Ts]  Denominator=[1 -1]  InitialStates=Q0  SampleTime=Ts
  y : Outport
  dy : Outport  Port=2
  wires:
  Discrete FIR Filter1/1 -> Discrete Filter/1, dy/1
  x/1 -> Discrete FIR Filter1/1
  Discrete Filter/1 -> y/1

== system TrajectoryGenerator2DOF_freq/Trajectory Generator9/M33 ==
  x : Inport
  Discrete FIR Filter1 : DiscreteFir  Coefficients=1/N/Ts*[1 zeros(1,N-1) -1]  InitialStates=Q0  SampleTime=Ts
  Discrete Filter : DiscreteFilter  Numerator=[0 Ts]  Denominator=[1 -1]  InitialStates=Q0  SampleTime=Ts
  y : Outport
  dy : Outport  Port=2
  wires:
  Discrete FIR Filter1/1 -> Discrete Filter/1, dy/1
  x/1 -> Discrete FIR Filter1/1
  Discrete Filter/1 -> y/1

== system TrajectoryGenerator2DOF_freq/Trajectory Generator9/M34 ==
  x : Inport
  Discrete FIR Filter1 : DiscreteFir  Coefficients=1/N/Ts*[1 zeros(1,N-1) -1]  InitialStates=Q0  SampleTime=Ts
  Discrete Filter : DiscreteFilter  Numerator=[0 Ts]  Denominator=[1 -1]  InitialStates=Q0  SampleTime=Ts
  y : Outport
  dy : Outport  Port=2
  wires:
  Discrete FIR Filter1/1 -> Discrete Filter/1, dy/1
  x/1 -> Discrete FIR Filter1/1
  Discrete Filter/1 -> y/1

== system TrajectoryGenerator2DOF_freq/Trajectory Generator9/M35 ==
  x : Inport
  Discrete FIR Filter1 : DiscreteFir  Coefficients=1/N/Ts*[1 zeros(1,N-1) -1]  InitialStates=Q0  SampleTime=Ts
  Discrete Filter : DiscreteFilter  Numerator=[0 Ts]  Denominator=[1 -1]  InitialStates=Q0  SampleTime=Ts
  y : Outport
  dy : Outport  Port=2
  wires:
  Discrete FIR Filter1/1 -> Discrete Filter/1, dy/1
  x/1 -> Discrete FIR Filter1/1
  Discrete Filter/1 -> y/1

== system TrajectoryGenerator2DOF_freq/Trajectory Generator9/M36 ==
  x : Inport
  Discrete FIR Filter1 : DiscreteFir  Coefficients=1/N/Ts*[1 zeros(1,N-1) -1]  InitialStates=Q0  SampleTime=Ts
  Discrete Filter : DiscreteFilter  Numerator=[0 Ts]  Denominator=[1 -1]  InitialStates=Q0  SampleTime=Ts
  y : Outport
  dy : Outport  Port=2
  wires:
  Discrete FIR Filter1/1 -> Discrete Filter/1, dy/1
  x/1 -> Discrete FIR Filter1/1
  Discrete Filter/1 -> y/1

== system TrajectoryGenerator2DOF_freq/Trajectory Generator9/M44 ==
  x : Inport
  Discrete FIR Filter1 : DiscreteFir  Coefficients=1/N/Ts*[1 zeros(1,N-1) -1]  InitialStates=Q0  SampleTime=Ts
  Discrete Filter : DiscreteFilter  Numerator=[0 Ts]  Denominator=[1 -1]  InitialStates=Q0  SampleTime=Ts
  y : Outport
  dy : Outport  Port=2
  wires:
  Discrete FIR Filter1/1 -> Discrete Filter/1, dy/1
  x/1 -> Discrete FIR Filter1/1
  Discrete Filter/1 -> y/1

== system TrajectoryGenerator2DOF_freq/Trajectory Generator9/M45 ==
  x : Inport
  Discrete FIR Filter1 : DiscreteFir  Coefficients=1/N/Ts*[1 zeros(1,N-1) -1]  InitialStates=Q0  SampleTime=Ts
  Discrete Filter : DiscreteFilter  Numerator=[0 Ts]  Denominator=[1 -1]  InitialStates=Q0  SampleTime=Ts
  y : Outport
  dy : Outport  Port=2
  wires:
  Discrete FIR Filter1/1 -> Discrete Filter/1, dy/1
  x/1 -> Discrete FIR Filter1/1
  Discrete Filter/1 -> y/1

== system TrajectoryGenerator2DOF_freq/Trajectory Generator9/M46 ==
  x : Inport
  Discrete FIR Filter1 : DiscreteFir  Coefficients=1/N/Ts*[1 zeros(1,N-1) -1]  InitialStates=Q0  SampleTime=Ts
  Discrete Filter : DiscreteFilter  Numerator=[0 Ts]  Denominator=[1 -1]  InitialStates=Q0  SampleTime=Ts
  y : Outport
  dy : Outport  Port=2
  wires:
  Discrete FIR Filter1/1 -> Discrete Filter/1, dy/1
  x/1 -> Discrete FIR Filter1/1
  Discrete Filter/1 -> y/1

== system TrajectoryGenerator2DOF_freq/Trajectory Generator9/M55 ==
  x : Inport
  Discrete FIR Filter1 : DiscreteFir  Coefficients=1/N/Ts*[1 zeros(1,N-1) -1]  InitialStates=Q0  SampleTime=Ts
  Discrete Filter : DiscreteFilter  Numerator=[0 Ts]  Denominator=[1 -1]  InitialStates=Q0  SampleTime=Ts
  y : Outport
  dy : Outport  Port=2
  wires:
  Discrete FIR Filter1/1 -> Discrete Filter/1, dy/1
  x/1 -> Discrete FIR Filter1/1
  Discrete Filter/1 -> y/1

== system TrajectoryGenerator2DOF_freq/Trajectory Generator9/M56 ==
  x : Inport
  Discrete FIR Filter1 : DiscreteFir  Coefficients=1/N/Ts*[1 zeros(1,N-1) -1]  InitialStates=Q0  SampleTime=Ts
  Discrete Filter : DiscreteFilter  Numerator=[0 Ts]  Denominator=[1 -1]  InitialStates=Q0  SampleTime=Ts
  y : Outport
  dy : Outport  Port=2
  wires:
  Discrete FIR Filter1/1 -> Discrete Filter/1, dy/1
  x/1 -> Discrete FIR Filter1/1
  Discrete Filter/1 -> y/1

== system TrajectoryGenerator2DOF_freq/Trajectory Generator9/M66 ==
  x : Inport
  Discrete FIR Filter1 : DiscreteFir  Coefficients=1/N/Ts*[1 zeros(1,N-1) -1]  InitialStates=Q0  SampleTime=Ts
  Discrete Filter : DiscreteFilter  Numerator=[0 Ts]  Denominator=[1 -1]  InitialStates=Q0  SampleTime=Ts
  y : Outport
  dy : Outport  Port=2
  wires:
  Discrete FIR Filter1/1 -> Discrete Filter/1, dy/1
  x/1 -> Discrete FIR Filter1/1
  Discrete Filter/1 -> y/1
